simulink model "May_26_HHD_Summer_v1_1"  (R2024b)
settings: Solver=ode45  StartTime=0.0  StopTime=672  MaxStep=.1  RelTol=1e-3  EnableMultiTasking=on
undefined symbols (not defined in the file): DC_CpS, DCHrS, HHDS, Hour, HPPS
libraries: slpidlib x2
settings Model: SimulationMode=accelerator  Creator=privotti  LastModifiedBy=peterknorth
settings SolverCC: AlgebraicLoopSolver=TrustRegion
settings DataIOCC: LimitDataPoints=on  SaveFormat=Array  ReturnWorkspaceOutputs=off  OutputOption=SpecifiedOutputTimes  OutputTimes=0:1:672
settings OptimizationCC: LifeSpan=inf
settings DebuggingCC: SolverPrmCheckMsg=warning  UnconnectedInputMsg=warning  UnconnectedOutputMsg=warning  UnconnectedLineMsg=warning  SFUnexpectedBacktrackingDiag=warning  SFNoUnconditionalDefaultTransitionDiag=warning  SFExecutionAtInitializationDiag=none  ArithmeticOperatorsInVariantConditions=warning
settings HardwareCC: ProdBitPerPointer=32  ProdBitPerSizeT=32  ProdBitPerPtrDiffT=32  ProdLargestAtomicFloat=None  ProdIntDivRoundTo=Undefined  ProdEndianess=Unspecified  ProdWordSize=32  ProdHWDeviceType=32-bit Generic
settings ModelReferenceCC: EnableRefExpFcnMdlSchedulingChecks=on  PropagateSignalLabelsOutOfModel=off
settings SFSimCC: SimUseLocalCustomCode=off  CustomCodeUndefinedFunction=UseInterfaceOnly
settings RTWCC: RTWUseLocalCustomCode=off  GPUComputeCapability=3.5
settings CodeAppCC: StateflowObjectComments=on
settings GRTTargetCC: TargetLangStandard=C89/C90 (ANSI)
settings ConfigComp: CovMetricSettings=dw  CovSaveCumulativeToWorkspaceVar=on  CovSaveSingleToWorkspaceVar=on  CovExternalEMLEnable=off  CovSFcnEnable=off

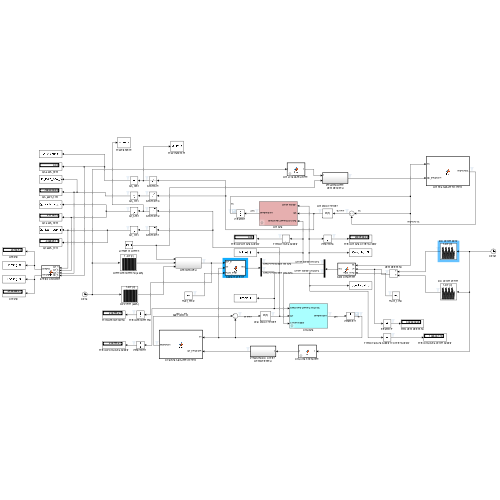
[thumbnail: Simulink's stored preview of the top-level diagram]
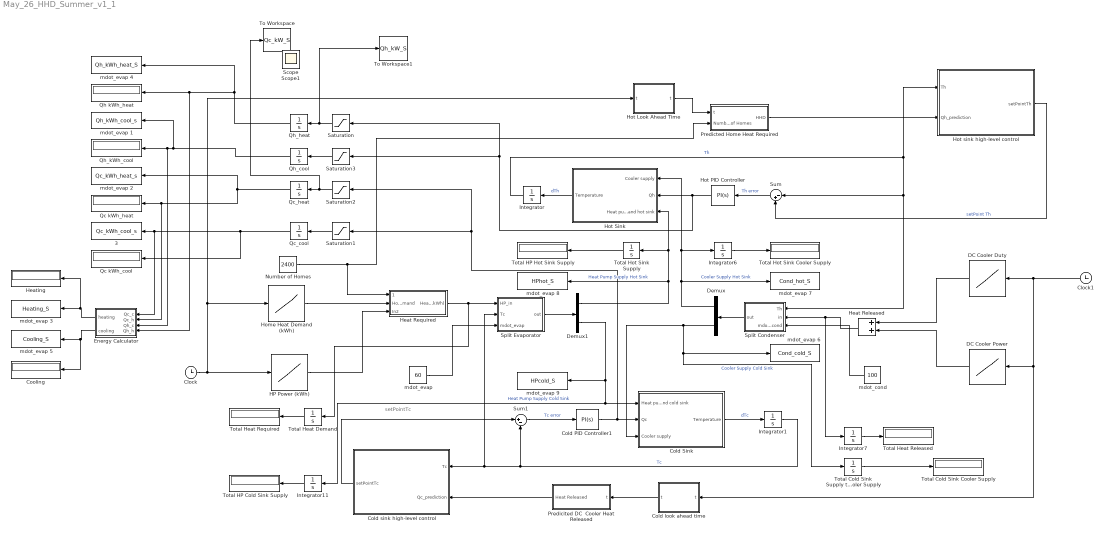
== system May_26_HHD_Summer_v1_1 ==
  note: setPointTc
  " Predicted Home Heat Required" : Subsystem  TreatAsAtomicUnit=on
  " Total HP Cold Sink Supply" : Display
      settings: Format=bank
  3 : ToWorkspace  VariableName=Qc_kWh_cool_s  SaveFormat=Timeseries  SampleTime=-1
  Clock : Clock
      settings: Decimation=100
  Clock1 : Clock
  Cold PID Controller1 : slpidlib/PID Controller  Controller=PI  Form=Parallel  TimeDomain=Continuous-time  UseExternalTs=off  SampleTime=-1  IntegratorMethod=Forward Euler  FilterMethod=Forward Euler  ControllerParametersSource=internal  P=26.5446187717975  I=15.3255427934333  UseKiTs=off  D=0  UseExternalDerivativeSource=off  N=0  UseFilter=on  TunerSelectOption=Transfer Function Based (PID Tuner App)  InitialConditionSource=internal  InitialConditionForIntegrator=1  InitialConditionForFilter=0  DifferentiatorICPrevScaledInput=0  ExternalReset=none  TrackingMode=off  Kt=1  LimitOutput=off  SatLimitsSource=internal  UpperSaturationLimit=70  LowerSaturationLimit=0  LinearizeAsGain=on  AntiWindupMode=clamping  Kb=1  LimitIntegrator=off  UpperIntegratorSaturationLimit=inf  LowerIntegratorSaturationLimit=-inf  POutMin=[]  POutMax=[]  IOutMin=[]  IOutMax=[]  DOutMin=[]  DOutMax=[]  NOutMin=[]  NOutMax=[]  SumOutMin=[]  SumOutMax=[]  SaturationOutMin=[]  SaturationOutMax=[]  PParamMin=[]  PParamMax=[]  IParamMin=[]  IParamMax=[]  DParamMin=[]  DParamMax=[]  NParamMin=[]  NParamMax=[]  KbParamMin=[]  KbParamMax=[]  KtParamMin=[]  KtParamMax=[]  KbOutMin=[]  KbOutMax=[]  KtOutMin=[]  KtOutMax=[]  IntegratorOutMin=[]  IntegratorOutMax=[]  FilterOutMin=[]  FilterOutMax=[]  SumI1OutMin=[]  SumI1OutMax=[]  SumI2OutMin=[]  SumI2OutMax=[]  SumI3OutMin=[]  SumI3OutMax=[]  SumI4OutMin=[]  SumI4OutMax=[]  SumDOutMin=[]  SumDOutMax=[]  DifferentiatorOutMin=[]  DifferentiatorOutMax=[]  FilterDiffOutCoefMin=[]  FilterDiffOutCoefMax=[]  ReciprocalOutMin=[]  ReciprocalOutMax=[]  SumDenOutMin=[]  SumDenOutMax=[]  SumNumOutMin=[]  SumNumOutMax=[]  DivideOutMin=[]  DivideOutMax=[]  UdiffTsProdOutMin=[]  UdiffTsProdOutMax=[]  NTsProdOutMin=[]  NTsProdOutMax=[]  UintegralTsProdOutMin=[]  UintegralTsProdOutMax=[]  UngainTsProdOutMin=[]  UngainTsProdOutMax=[]  ClampingZeroOutDataTypeStr=Inherit: Inherit via back propagation  ClampingZeroOutMin=[]  ClampingZeroOutMax=[]  FilterDenConstantOutDataTypeStr=Inherit: Inherit via back propagation  FilterDenConstantOutMin=[]  FilterDenConstantOutMax=[]  PCopyOutDataTypeStr=Inherit: Inherit via back propagation  PCopyOutMin=[]  PCopyOutMax=[]  NCopyOutDataTypeStr=Inherit: Inherit via back propagation  NCopyOutMin=[]  NCopyOutMax=[]  IntegratorContinuousStateAttributes=''  IntegratorStateMustResolveToSignalObject=off  IntegratorRTWStateStorageClass=Auto  FilterContinuousStateAttributes=''  FilterStateMustResolveToSignalObject=off  FilterRTWStateStorageClass=Auto  ParallelPVariant=InternalParameters  IdealPVariant=Disabled  IVariant=InternalParameters  DVariant=Disabled  IntegratorVariant=Continuous  SatVariant=Disabled  AWVariant=Passthrough  PCopyVariant=Disabled  TRVariant=Disabled  FdbkBlocksVariant=Forward  IdealPFdbkVariant=Disabled  SatFdbkVariant=Disabled  DerivativeFilterVariant=Disabled  NVariant=Disabled  NCopyVariant=Disabled_SignalSpec  FilterICVariant=Disabled  IntegratorICVariant=InternalICs  ExternalResetVariant=Disabled  TRSumVariant=Passthrough  SumFdbkVariant=Disabled  SumVariant=Sum_PI  TsampFilterVariant=InternalTs  TsampNgainVariant=Passthrough  TsampIntegralVariant=Disabled_SignalSpec  ExternalSaturationOutDataTypeStr=Inherit: Same as second input  DerivativeSourceVariant=Disabled  PreIntVariant=InternalPreInt
  Cold Sink : Subsystem  mask{TargetTemperature=10}
      mask prompts: TargetTemperature "Target temperature"
  Cold look ahead time : MATLAB Function  TreatAsAtomicUnit=on  mask{hoursToLookAhead=0.1}
      mask prompts: hoursToLookAhead "Hours to look ahead"
  Cold sink high-level control : MATLAB Function  TreatAsAtomicUnit=on
  Cooling : Display
      settings: Format=bank
  DC Cooler Duty : Lookup_n-D  NumberOfTableDimensions=1  BreakpointsForDimension1=Hour  Table=DCHrS  InternalRulePriority=Speed  RndMeth=Simplest
  DC Cooler Power : Lookup_n-D  NumberOfTableDimensions=1  BreakpointsForDimension1=Hour  Table=DC_CpS  InternalRulePriority=Speed  RndMeth=Simplest
  Demux : Demux  Outputs=2
  Demux1 : Demux  Outputs=2
  Energy Calculator : MATLAB Function  TreatAsAtomicUnit=on
  HP Power (kWh) : Lookup_n-D  NumberOfTableDimensions=1  BreakpointsForDimension1=Hour  Table=HPPS  InternalRulePriority=Speed  RndMeth=Simplest
  Heat Released : Sum
  Heat Required : Subsystem
  Heating : Display
      settings: Format=bank
  Home Heat Demand (kWh) : Lookup_n-D  NumberOfTableDimensions=1  BreakpointsForDimension1=Hour  Table=HHDS  InternalRulePriority=Speed  RndMeth=Simplest
  "Hot Look Ahead Time " : MATLAB Function  TreatAsAtomicUnit=on  mask{hoursToLookAhead=0.1}
      mask prompts: hoursToLookAhead "Hours to look ahead"
  Hot PID Controller : slpidlib/PID Controller  Controller=PI  Form=Parallel  TimeDomain=Continuous-time  UseExternalTs=off  SampleTime=-1  IntegratorMethod=Forward Euler  FilterMethod=Forward Euler  ControllerParametersSource=internal  P=392.15264275082  I=1.05921801558609  UseKiTs=off  D=0  UseExternalDerivativeSource=off  N=0  UseFilter=on  TunerSelectOption=Transfer Function Based (PID Tuner App)  InitialConditionSource=internal  InitialConditionForIntegrator=-1  InitialConditionForFilter=0  DifferentiatorICPrevScaledInput=0  ExternalReset=none  TrackingMode=off  Kt=1  LimitOutput=off  SatLimitsSource=internal  UpperSaturationLimit=50  LowerSaturationLimit=0  LinearizeAsGain=on  AntiWindupMode=clamping  Kb=1  LimitIntegrator=off  UpperIntegratorSaturationLimit=inf  LowerIntegratorSaturationLimit=-inf  POutMin=[]  POutMax=[]  IOutMin=[]  IOutMax=[]  DOutMin=[]  DOutMax=[]  NOutMin=[]  NOutMax=[]  SumOutMin=[]  SumOutMax=[]  SaturationOutMin=[]  SaturationOutMax=[]  PParamMin=[]  PParamMax=[]  IParamMin=[]  IParamMax=[]  DParamMin=[]  DParamMax=[]  NParamMin=[]  NParamMax=[]  KbParamMin=[]  KbParamMax=[]  KtParamMin=[]  KtParamMax=[]  KbOutMin=[]  KbOutMax=[]  KtOutMin=[]  KtOutMax=[]  IntegratorOutMin=[]  IntegratorOutMax=[]  FilterOutMin=[]  FilterOutMax=[]  SumI1OutMin=[]  SumI1OutMax=[]  SumI2OutMin=[]  SumI2OutMax=[]  SumI3OutMin=[]  SumI3OutMax=[]  SumI4OutMin=[]  SumI4OutMax=[]  SumDOutMin=[]  SumDOutMax=[]  DifferentiatorOutMin=[]  DifferentiatorOutMax=[]  FilterDiffOutCoefMin=[]  FilterDiffOutCoefMax=[]  ReciprocalOutMin=[]  ReciprocalOutMax=[]  SumDenOutMin=[]  SumDenOutMax=[]  SumNumOutMin=[]  SumNumOutMax=[]  DivideOutMin=[]  DivideOutMax=[]  UdiffTsProdOutMin=[]  UdiffTsProdOutMax=[]  NTsProdOutMin=[]  NTsProdOutMax=[]  UintegralTsProdOutMin=[]  UintegralTsProdOutMax=[]  UngainTsProdOutMin=[]  UngainTsProdOutMax=[]  ClampingZeroOutDataTypeStr=Inherit: Inherit via back propagation  ClampingZeroOutMin=[]  ClampingZeroOutMax=[]  FilterDenConstantOutDataTypeStr=Inherit: Inherit via back propagation  FilterDenConstantOutMin=[]  FilterDenConstantOutMax=[]  PCopyOutDataTypeStr=Inherit: Inherit via back propagation  PCopyOutMin=[]  PCopyOutMax=[]  NCopyOutDataTypeStr=Inherit: Inherit via back propagation  NCopyOutMin=[]  NCopyOutMax=[]  IntegratorContinuousStateAttributes=''  IntegratorStateMustResolveToSignalObject=off  IntegratorRTWStateStorageClass=Auto  FilterContinuousStateAttributes=''  FilterStateMustResolveToSignalObject=off  FilterRTWStateStorageClass=Auto  ParallelPVariant=InternalParameters  IdealPVariant=Disabled  IVariant=InternalParameters  DVariant=Disabled  IntegratorVariant=Continuous  SatVariant=Disabled  AWVariant=Passthrough  PCopyVariant=Disabled  TRVariant=Disabled  FdbkBlocksVariant=Forward  IdealPFdbkVariant=Disabled  SatFdbkVariant=Disabled  DerivativeFilterVariant=Disabled  NVariant=Disabled  NCopyVariant=Disabled_SignalSpec  FilterICVariant=Disabled  IntegratorICVariant=InternalICs  ExternalResetVariant=Disabled  TRSumVariant=Passthrough  SumFdbkVariant=Disabled  SumVariant=Sum_PI  TsampFilterVariant=InternalTs  TsampNgainVariant=Passthrough  TsampIntegralVariant=Disabled_SignalSpec  ExternalSaturationOutDataTypeStr=Inherit: Same as second input  DerivativeSourceVariant=Disabled  PreIntVariant=InternalPreInt
  Hot Sink : Subsystem  mask{initialTemperature=20}
      mask prompts: initialTemperature "Initial temperature"
  Hot sink high-level control : MATLAB Function  TreatAsAtomicUnit=on
  Integrator : Integrator  InitialCondition=20
  Integrator1 : Integrator  InitialCondition=10
  Integrator11 : Integrator
  Integrator6 : Integrator
  Integrator7 : Integrator
  Number of Homes : Constant  Value=2400
  Predicited DC  Cooler Heat Released : Subsystem  TreatAsAtomicUnit=on
  Qc kWh_cool : Display
      settings: Format=bank
  Qc kWh_heat : Display
      settings: Format=bank
  Qc_cool : Integrator
  Qc_heat : Integrator
  Qh kWh_heat : Display
      settings: Format=bank
  Qh_cool : Integrator
  Qh_heat : Integrator
  Qh_kWh_cool : Display
      settings: Format=bank
  Saturation : Saturate  UpperLimit=inf  LowerLimit=0
  Saturation1 : Saturate  UpperLimit=0  LowerLimit=-inf
  Saturation2 : Saturate  UpperLimit=inf  LowerLimit=0
  Saturation3 : Saturate  UpperLimit=0  LowerLimit=-inf
  Split Condenser : MATLAB Function  TreatAsAtomicUnit=on
  Split Evaporator : MATLAB Function  TreatAsAtomicUnit=on
  Sum : Sum  Inputs=|-+
  Sum1 : Sum  Inputs=|+-
  To Workspace : ToWorkspace  VariableName=Qc_kW_S  SampleTime=-1
      settings: Save2DSignal=2-D array (concatenate along first dimension)
  To Workspace1 : ToWorkspace  VariableName=Qh_kW_S  SampleTime=-1
      settings: Save2DSignal=2-D array (concatenate along first dimension)
  Total Cold Sink Cooler Supply : Display
      settings: Format=bank
  Total Cold Sink Supply to Cooler Supply : Integrator
  Total HP Hot Sink Supply : Display
      settings: Format=bank
  Total Heat Demand : Integrator
  Total Heat Released : Display
      settings: Format=bank
  Total Heat Required : Display
      settings: Format=bank
  Total Hot Sink Cooler Supply : Display
      settings: Format=bank
  Total Hot Sink Supply : Integrator
  mdot_cond : Constant  Value=100  VectorParams1D=off
  mdot_evap : Constant  Value=60  VectorParams1D=off
  mdot_evap 1 : ToWorkspace  VariableName=Qh_kWh_cool_s  SaveFormat=Timeseries  SampleTime=-1
  mdot_evap 2 : ToWorkspace  VariableName=Qc_kWh_heat_s  SaveFormat=Timeseries  SampleTime=-1
  mdot_evap 3 : ToWorkspace  VariableName=Heating_S  SaveFormat=Timeseries  SampleTime=-1
  mdot_evap 4 : ToWorkspace  VariableName=Qh_kWh_heat_S  SaveFormat=Timeseries  SampleTime=-1
  mdot_evap 5 : ToWorkspace  VariableName=Cooling_S  SaveFormat=Timeseries  SampleTime=-1
  mdot_evap 6 : ToWorkspace  VariableName=Cond_cold_S  SaveFormat=Timeseries  SampleTime=-1
  mdot_evap 7 : ToWorkspace  VariableName=Cond_hot_S  SaveFormat=Timeseries  SampleTime=-1
  mdot_evap 8 : ToWorkspace  VariableName=HPhot_S  SaveFormat=Timeseries  SampleTime=-1
  mdot_evap 9 : ToWorkspace  VariableName=HPcold_S  SaveFormat=Timeseries  SampleTime=-1
  Scope : Scope
  Scope1 : Scope
  wires:
  Demux/1 -> mdot_evap 7/1, Integrator6/1, Hot Sink/1("Cooler supply ")  "Cooler Supply Hot Sink"
  Demux1/1 -> mdot_evap 8/1, Total Hot Sink Supply/1, Hot Sink/3(Heat pump demand hot sink)  "Heat Pump Supply Hot Sink"
  Demux1/2 -> mdot_evap 9/1, Cold Sink/1(Heat pump demand cold sink), Integrator11/1  "Heat Pump Supply Cold Sink"
  Demux/2 -> mdot_evap 6/1, Total Cold Sink Supply to Cooler Supply/1, Cold Sink/3(Cooler supply)  "Cooler Supply Cold Sink"
  Hot Sink/1(Temperature) -> Integrator/1  "dTh"
  Cold Sink/1(Temperature) -> Integrator1/1  "dTc"
  Hot PID Controller/1 -> Saturation3/1, Saturation/1, Hot Sink/2(Qh)
  Sum/1 -> Hot PID Controller/1  "Th error"
  Cold sink high-level control/1(setPointTc) -> Sum1/1
  Sum1/1 -> Cold PID Controller1/1  "Tc error"
  Hot sink high-level control/1(setPointTh) -> Sum/2  "setPoint Th"
  Clock/1 -> HP Power (kWh)/1, Home Heat Demand (kWh)/1, "Hot Look Ahead Time "/1("t ")
  Integrator/1 -> Hot sink high-level control/1(Th), Sum/1, Split Condenser/1(Th)  "Th"
  Integrator1/1 -> Split Evaporator/2(Tc), Cold sink high-level control/1(Tc), Sum1/2  "Tc"
  Split Condenser/1(out) -> Demux/1
  Split Evaporator/1(out) -> Demux1/1
  HP Power (kWh)/1 -> Heat Required/3(In2)
  " Predicted Home Heat Required"/1(HHD) -> Hot sink high-level control/2(Qh_prediction)
  Predicited DC  Cooler Heat Released/1(Heat Released) -> Cold sink high-level control/2(Qc_prediction)
  Clock1/1 -> Cold look ahead time/1("t "), DC Cooler Power/1, DC Cooler Duty/1
  Cold look ahead time/1(t) -> Predicited DC  Cooler Heat Released/1(t)
  "Hot Look Ahead Time "/1(t) -> " Predicted Home Heat Required"/1(t)
  DC Cooler Duty/1 -> Heat Released/1
  DC Cooler Power/1 -> Heat Released/2
  Heat Released/1 -> Split Condenser/2(in), Integrator7/1
  Home Heat Demand (kWh)/1 -> Heat Required/2(Home Heat Demand)
  Number of Homes/1 -> " Predicted Home Heat Required"/2(Number of Homes), Heat Required/1(" ")
  Heat Required/1("Heat Required (kWh)  ") -> Total Heat Demand/1, Split Evaporator/1(HP_in)
  mdot_cond/1 -> Split Condenser/3(mdot_cond)
  mdot_evap/1 -> Split Evaporator/3(mdot_evap)
  Cold PID Controller1/1 -> Saturation2/1, Saturation1/1, Cold Sink/2(Qc)
  Saturation2/1 -> To Workspace/1, Qc_heat/1
  Saturation1/1 -> Qc_cool/1
  Qc_heat/1 -> mdot_evap 2/1, Energy Calculator/2(Qc_h), Qc kWh_heat/1
  Saturation3/1 -> Qh_cool/1
  Saturation/1 -> To Workspace1/1, Qh_heat/1
  Qc_cool/1 -> Energy Calculator/1(Qc_c), 3/1, Qc kWh_cool/1
  Qh_cool/1 -> Qh_kWh_cool/1, Energy Calculator/3(Qh_c), mdot_evap 1/1
  Qh_heat/1 -> mdot_evap 4/1, Energy Calculator/4(Qh_h), Qh kWh_heat/1
  Integrator6/1 -> Total Hot Sink Cooler Supply/1
  Total Cold Sink Supply to Cooler Supply/1 -> Total Cold Sink Cooler Supply/1
  Integrator7/1 -> Total Heat Released/1
  Total Hot Sink Supply/1 -> Total HP Hot Sink Supply/1
  Integrator11/1 -> " Total HP Cold Sink Supply"/1
  Total Heat Demand/1 -> Total Heat Required/1
  Energy Calculator/1(heating) -> Heating/1, mdot_evap 3/1
  Energy Calculator/2(cooling) -> Cooling/1, mdot_evap 5/1

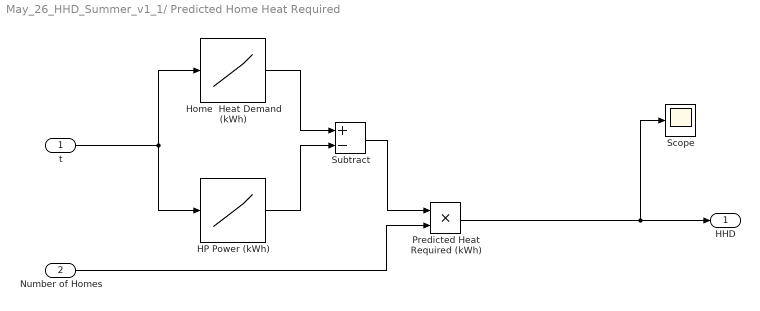
== system May_26_HHD_Summer_v1_1/ Predicted Home Heat Required ==
  t : Inport
  Number of Homes : Inport  Port=2
  HP Power (kWh) : Lookup_n-D  NumberOfTableDimensions=1  BreakpointsForDimension1=Hour  Table=HPPS  InternalRulePriority=Speed  RndMeth=Simplest
  Home  Heat Demand (kWh) : Lookup_n-D  NumberOfTableDimensions=1  BreakpointsForDimension1=Hour  Table=HHDS  InternalRulePriority=Speed  RndMeth=Simplest
  Predicted Heat Required (kWh) : Product
  Scope : Scope
  Subtract : Sum  Inputs=+-
  HHD : Outport
  wires:
  t/1 -> HP Power (kWh)/1, Home  Heat Demand (kWh)/1
  HP Power (kWh)/1 -> Subtract/2
  Number of Homes/1 -> Predicted Heat Required (kWh)/2
  Subtract/1 -> Predicted Heat Required (kWh)/1
  Predicted Heat Required (kWh)/1 -> HHD/1, Scope/1
  Home  Heat Demand (kWh)/1 -> Subtract/1

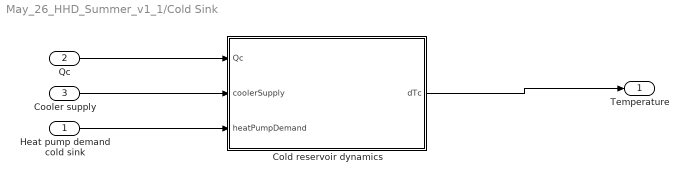
== system May_26_HHD_Summer_v1_1/Cold Sink ==
  Heat pump demand cold sink : Inport
  Qc : Inport  Port=2
  Cooler supply : Inport  Port=3
  Cold reservoir dynamics : MATLAB Function  TreatAsAtomicUnit=on
  Temperature : Outport  VectorParamsAs1DForOutWhenUnconnected=off
  wires:
  Cooler supply/1 -> Cold reservoir dynamics/2(coolerSupply)
  Qc/1 -> Cold reservoir dynamics/1(Qc)
  Heat pump demand cold sink/1 -> Cold reservoir dynamics/3(heatPumpDemand)
  Cold reservoir dynamics/1(dTc) -> Temperature/1

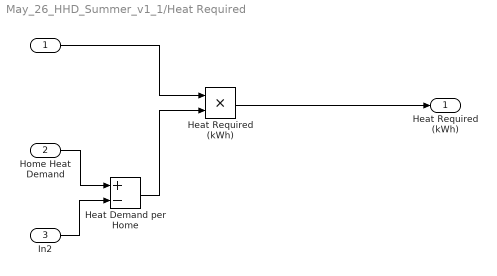
== system May_26_HHD_Summer_v1_1/Heat Required ==
  " " : Inport
  Home Heat Demand : Inport  Port=2
  In2 : Inport  Port=3
  "Heat Demand per Home " : Sum  Inputs=+-
  Heat Required (kWh) : Product
  "Heat Required (kWh)  " : Outport
  wires:
  Home Heat Demand/1 -> "Heat Demand per Home "/1
  "Heat Demand per Home "/1 -> Heat Required (kWh)/2
  In2/1 -> "Heat Demand per Home "/2
  " "/1 -> Heat Required (kWh)/1
  Heat Required (kWh)/1 -> "Heat Required (kWh)  "/1

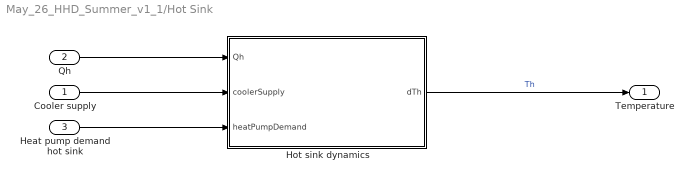
== system May_26_HHD_Summer_v1_1/Hot Sink ==
  "Cooler supply " : Inport
  Qh : Inport  Port=2
  Heat pump demand hot sink : Inport  Port=3
  Hot sink dynamics : MATLAB Function  TreatAsAtomicUnit=on
  Temperature : Outport  VectorParamsAs1DForOutWhenUnconnected=off
  wires:
  "Cooler supply "/1 -> Hot sink dynamics/2(coolerSupply)
  Qh/1 -> Hot sink dynamics/1(Qh)
  Heat pump demand hot sink/1 -> Hot sink dynamics/3(heatPumpDemand)
  Hot sink dynamics/1(dTh) -> Temperature/1  "Th"

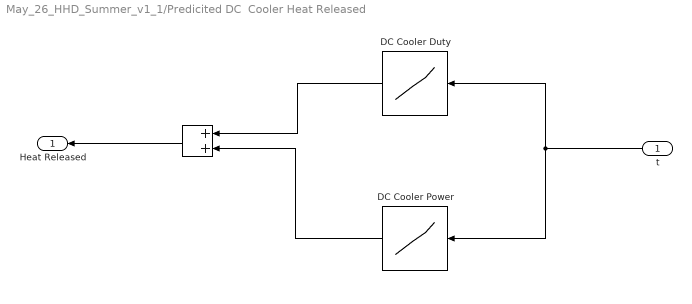
== system May_26_HHD_Summer_v1_1/Predicited DC  Cooler Heat Released ==
  t : Inport
  "  " : Sum
  DC Cooler Duty : Lookup_n-D  NumberOfTableDimensions=1  BreakpointsForDimension1=Hour  Table=DCHrS  InternalRulePriority=Speed  RndMeth=Simplest
  DC Cooler Power : Lookup_n-D  NumberOfTableDimensions=1  BreakpointsForDimension1=Hour  Table=DC_CpS  InternalRulePriority=Speed  RndMeth=Simplest
  Heat Released : Outport
  wires:
  t/1 -> DC Cooler Duty/1, DC Cooler Power/1
  DC Cooler Power/1 -> "  "/2
  DC Cooler Duty/1 -> "  "/1
  "  "/1 -> Heat Released/1

== matlab function May_26_HHD_Summer_v1_1/Split Evaporator ==
  data: HP_in input; out output; Tc input; mdot_evap input
function out = fcn(HP_in, Tc, mdot_evap)
%#codegen
% Calculates the split of heat supply to the HP evaporator 
% from the hot and cold sinks based on the cold sink
% temperate and heat that can be transfered, with the remaining heat coming from to the hot sink 
% If beta > in, beta limited to in and all heat goes to evaporator
% condenser

e = 0.9;        % evaporator effectiveness
Thp = 5;        % HP evaporating temperature
cp = 4.18;      % specific heat of water [kJ/kg·K]
Cmin = cp * mdot_evap; % minimum heat transfer rate


beta = e * Cmin * (Tc - Thp); % heat from cold sink 

if beta > HP_in
    beta = HP_in;
    out = [0,beta];
else
    out = [HP_in - beta, beta]; % heat from (hot sink, cold sink)
end

== matlab function May_26_HHD_Summer_v1_1/Split Condenser ==
  data: Th input; out output; in input; mdot_cond input
function out = fcn(Th,in,mdot_cond)
%#codegen
% Calculates the split of heat supply released from the chiller condenser 
% to the hot and cold sinks based on the hot sink
% temperate and heat that can be transfered, with the remaining heat going to the cold sink 
% If alpha > in, alpha limited to in and all heat goes to hot sink

e = 0.9; % e = condenser effectiveness, using a preliminary design value.

cp = 4.18; % specific heat of water, kJ/kg·K

Cmin = cp * mdot_cond; % Minium heat transfer rate

Tcooler = 30; % chiller condensing temperature

alpha = e * Cmin * (Tcooler - Th); % heat to hot sink

if alpha > in
    alpha = in;
    out = [alpha,0];
else
    out = [alpha,in-alpha]; % heat to hot sink,cold sink
end

== matlab function May_26_HHD_Summer_v1_1/Hot Sink/Hot sink dynamics ==
  data: Qh input; dTh output; coolerSupply input; heatPumpDemand input
function dTh = fcn(Qh, coolerSupply, heatPumpDemand)
%#codegen

M = 40000; % thermal store mass, kg
Cp = 4.18; % Cp water kJ/(kg.K);
dTh = (Qh + coolerSupply - heatPumpDemand) / (M * Cp);

== matlab function May_26_HHD_Summer_v1_1/Cold Sink/Cold reservoir dynamics ==
  data: Qc input; dTc output; coolerSupply input; heatPumpDemand input
function dTc = fcn(Qc, coolerSupply, heatPumpDemand)
%#coegen
M = 40000; % thermal store mass, kg
Cp = 4.18; % specific heat water, kJ/(kg.K)

dTc = (coolerSupply - heatPumpDemand + Qc) / (M * Cp);

== matlab function May_26_HHD_Summer_v1_1/Hot sink high-level control ==
  settings: updateMethod=DISCRETE
  data: Th input; setPointTh output; Qh_prediction input
function setPointTh = fcn(Th,Qh_prediction)

%#codegen
% Rule-based temperature control with early return for small Th changes.
% If sink temperature change is less than 0.1°C, the function holds the
% previous set point and ignores any Qh_prediction updates.

persistent prevSetPointTh prevTh
if isempty(prevSetPointTh)
    prevSetPointTh = 20.0;   % initial setpoint
    prevTh = Th;             % initial temperature
end

% No-update logic: small change in Th → return immediately
if abs(Th - prevTh) < 0.1
    setPointTh = prevSetPointTh;
    return
end

% Rule-based logic
status = 'LL';

if Th < 20
    status(1) = 'L';
else
    status(1) = 'H';
end

if Qh_prediction < 500   % threshold for low heat load
    status(2) = 'L';
else
    status(2) = 'H';
end

switch status
    case 'LL'
        setPointTh = 22.0;
    case 'LH'
        setPointTh = 21.0;
    case 'HL'
        setPointTh = 19.0;
    case 'HH'
        setPointTh = 18.0;        
    otherwise
        setPointTh = 20; 
end

% Store current values for next call
prevSetPointTh = setPointTh;
prevTh = Th;

== matlab function May_26_HHD_Summer_v1_1/Energy Calculator ==
  data: Qc_c input; heating output; Qc_h input; Qh_c input; Qh_h input; cooling output
function [heating, cooling] = fcn(Qc_c, Qc_h, Qh_c, Qh_h)
%#codegen
vals = [Qc_c, Qc_h, Qh_c, Qh_h];
heating = sum(vals(vals > 0));
cooling = sum(vals(vals < 0));
end

== matlab function May_26_HHD_Summer_v1_1/Hot Look Ahead Time  ==
  data: t input; t output; hoursToLookAhead parameter
function t  = fcn(t, hoursToLookAhead)
t = mod(t + hoursToLookAhead,672);

== matlab function May_26_HHD_Summer_v1_1/Cold look ahead time ==
  data: t input; t output; hoursToLookAhead parameter
function t = fcn(t, hoursToLookAhead)
t = mod(t + hoursToLookAhead,672);

== matlab function May_26_HHD_Summer_v1_1/Cold sink high-level control ==
  settings: updateMethod=DISCRETE
  data: Tc input; setPointTc output; Qc_prediction input
function setPointTc = fcn(Tc, Qc_prediction)
%#codegen
% Rule-based temperature control with early return for small Tc changes.
% If sink temperature change is below 0.1°C, the function holds the
% previous set point and ignores any Qc_prediction updates.

persistent prevSetPointTc prevTc
if isempty(prevSetPointTc)
    prevSetPointTc = 10.0;   % initial setpoint
    prevTc = Tc;             % initial temperature
end

% No-update logic: small change in Tc → return immediately
if abs(Tc - prevTc) < 0.1
    setPointTc = prevSetPointTc;
    return
end

% rule-based logic
status = 'LL';

if Tc < 10
    status(1) = 'L';
else
    status(1) = 'H';
end

if Qc_prediction < 2500   % threshold for low heat load
    status(2) = 'L';
else
    status(2) = 'H';
end

switch status
    case 'LL'
        setPointTc = 12.0;
    case 'LH'
        setPointTc = 11.0;
    case 'HL'
        setPointTc = 9.0;
    case 'HH'
        setPointTc = 8.0;
    otherwise
        setPointTc = 10.0;
end

% Store current values for next call
prevSetPointTc = setPointTc;
prevTc = Tc;
